simulink model "Q11_2_SIM"  (R2024b)
settings: Solver=VariableStepAuto  StartTime=0.0  StopTime=10.0  RelTol=1e-3
values from neighbouring files (symbols this model uses):
  A_aug = [A zeros(5,1) ... (first row only)    [main.m]    (also in main_sim.m)
  B_aug = [B; 0]    [main.m]    (also in main_sim.m)
  C_aug = [C zeros(2,1)]    [main.m]    (also in main_sim.m)
  D = zeros(2,1)    [main.m]
  dead_zone_half_width = 0.2    [main.m]    (also in main_sim.m)
  K_aug = lqr(A_aug, B_aug, Qr, Rr)    [main.m]
  L_aug = [L ... (first row only)    [main.m]    (also in main_sim.m)
  x0 = [alpha_init 0 beta_init 0 0]'    [main.m]    (also in main_sim.m = [alpha_init 0 beta_init 0 0])
undefined symbols (not defined in the file or in its folder): A, B, C
libraries: simulink_extras x1
settings Model: Creator=pedro  LastModifiedBy=pedro

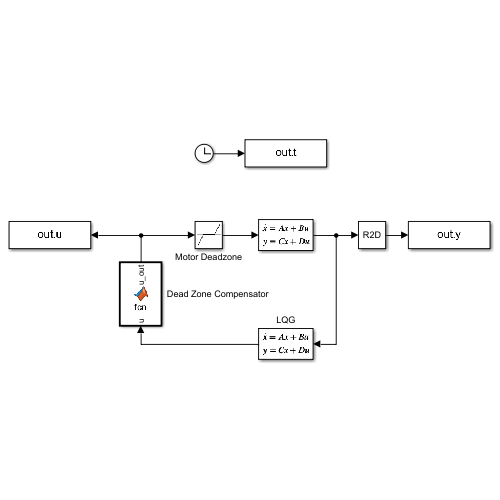
[thumbnail: Simulink's stored preview of the top-level diagram]
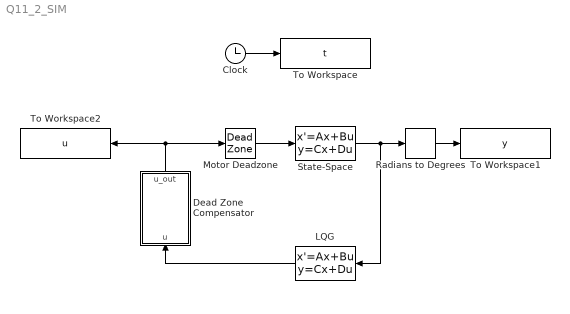
== system Q11_2_SIM ==
  Clock : Clock
  Dead Zone Compensator : MATLAB Function  TreatAsAtomicUnit=on
  LQG : StateSpace  A=A_aug - B_aug * K_aug - L_aug * C_aug  B=L_aug  C=-K_aug  D=zeros(1,2)  InitialCondition=0
  Motor Deadzone : DeadZone  LowerValue=-dead_zone_half_width  UpperValue=dead_zone_half_width
  Radians to Degrees : simulink_extras/Transformations/Radians to Degrees
  State-Space : StateSpace  A=A  B=B  C=C  D=D  InitialCondition=x0
  To Workspace : ToWorkspace  VariableName=t  SaveFormat=Timeseries  SampleTime=-1
  To Workspace1 : ToWorkspace  VariableName=y  SaveFormat=Timeseries  SampleTime=-1
  To Workspace2 : ToWorkspace  VariableName=u  SaveFormat=Timeseries  SampleTime=-1
  wires:
  Clock/1 -> To Workspace/1
  Dead Zone Compensator/1(u_out) -> To Workspace2/1, Motor Deadzone/1
  LQG/1 -> Dead Zone Compensator/1(u)
  Radians to Degrees/1 -> To Workspace1/1
  State-Space/1 -> Radians to Degrees/1, LQG/1
  Motor Deadzone/1 -> State-Space/1

== matlab function Q11_2_SIM/Dead Zone Compensator ==
  data: u input; u_out output
function u_out = fcn(u) 
    if u>0
        u_out= u + 0.2;
    elseif u<0
        u_out= u - 0.2;
    else 
        u_out = u;
    end
end
